simulink library "db_pino_crem_"  (R2014b)
settings: Solver=ode45  SolverMode=SingleTasking  StartTime=0.0  StopTime=10.0  RelTol=1e-3
values from neighbouring files (symbols this model uses):
  B1 = 40    [ejemplo_mecanico.m]    (also in veengranes.m = 10)
  B2 = 20    [ejemplo_mecanico.m]    (also in veengranes.m = 34)
  J = 12    [ejercicio7_taller2SM.m]    (also in motord_DC_rot.m = 0.01)
  M = 20    [Problem_5_Matlab.m]    (also in ejercicio7_taller2SM.m = 10; grupo_roberto.m = 1)
  R = 10    [anexo_parcial.m]    (also in ejemplo_electrico.m = 1000; ejercicio7_taller2SM.m = 0.01; motord_DC_rot.m; nivel_tanque.m = 37)
undefined symbols (not defined in the file or in its folder): K
settings Model: CovMetricSettings=dwe  CovHtmlReporting=off  CovSaveCumulativeToWorkspaceVar=off  CovSaveSingleToWorkspaceVar=off  CovExternalEMLEnable=on  CovSFcnEnable=on  Creator=carma  LastModifiedBy=carma

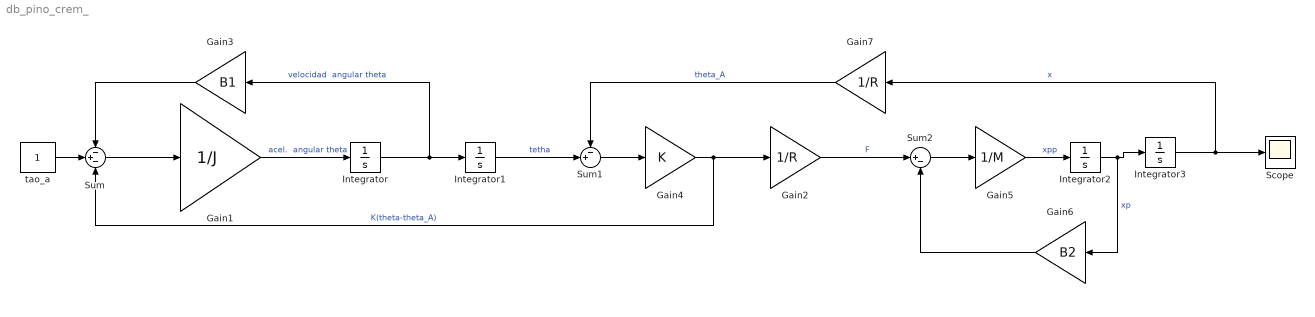
== system db_pino_crem_ ==
  Gain1 : Gain  Gain=1/J
  Gain2 : Gain  Gain=1/R
  Gain3 : Gain  Gain=B1
  Gain4 : Gain  Gain=K
  Gain5 : Gain  Gain=1/M
  Gain6 : Gain  Gain=B2
  Gain7 : Gain  Gain=1/R
  Integrator{,1..3} (4 alike) : Integrator
  Scope : Scope
      settings: TimeRange=auto  MaxDataPoints=5000  SaveToWorkspace=off  SaveName=ScopeData  YMin=-10  YMax=10  SampleTime=-1
  Sum : Sum  Inputs=-+-
  Sum1 : Sum  Inputs=-+|
  Sum2 : Sum  Inputs=|+-
  tao_a : Constant
  wires:
  Sum/1 -> Gain1/1
  Gain1/1 -> Integrator/1  "acel.  angular theta"
  Integrator/1 -> Gain3/1, Integrator1/1  "velocidad  angular theta"
  tao_a/1 -> Sum/2
  Gain3/1 -> Sum/1
  Sum1/1 -> Gain4/1
  Gain4/1 -> Sum/3, Gain2/1  "K(theta-theta_A)"
  Gain2/1 -> Sum2/1  "F"
  Integrator1/1 -> Sum1/2  "tetha"
  Gain7/1 -> Sum1/1  "theta_A"
  Sum2/1 -> Gain5/1
  Gain5/1 -> Integrator2/1  "xpp"
  Integrator2/1 -> Gain6/1, Integrator3/1  "xp"
  Integrator3/1 -> Gain7/1, Scope/1  "x"
  Gain6/1 -> Sum2/2
